simulink model "Quadcopter_Control_PID_Block_Updated"  (R2023a)
settings: Solver=VariableStepAuto  StartTime=0.0  StopTime=10.0  RelTol=1e-3
undefined symbols (not defined in the file or in its folder): sigbuilder_block
libraries: slpidlib x4
settings Model: Creator=Hameed  LastModifiedBy=Hameed
settings DebuggingCC: UnconnectedInputMsg=warning  UnconnectedOutputMsg=warning  UnconnectedLineMsg=warning
settings ModelReferenceCC: EnableRefExpFcnMdlSchedulingChecks=on
settings RTWCC: DLArmComputeVersion=19.05

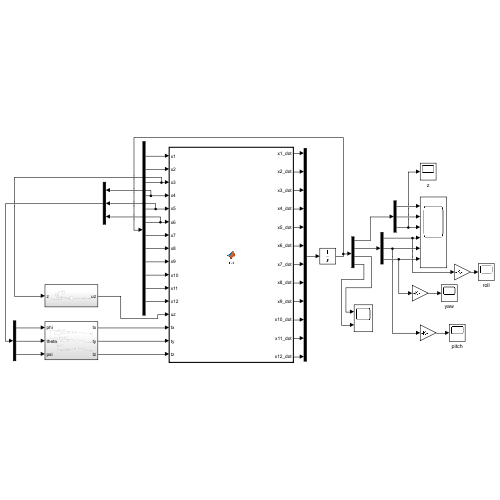
[thumbnail: Simulink's stored preview of the top-level diagram]
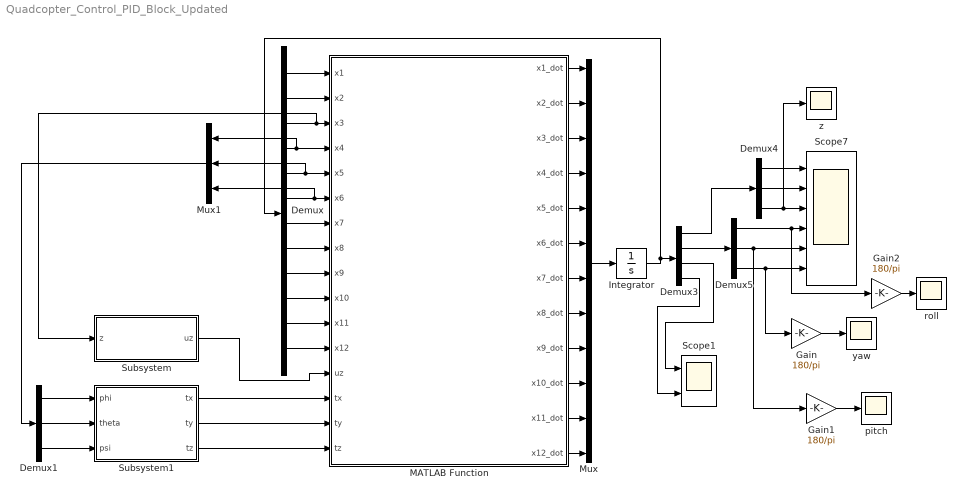
== system Quadcopter_Control_PID_Block_Updated ==
  Demux : Demux  Outputs=12
  Demux1 : Demux  Outputs=3
  Demux3 : Demux
  Demux4 : Demux  Outputs=3
  Demux5 : Demux  Outputs=3
  Gain : Gain  Gain=180/pi
  Gain1 : Gain  Gain=180/pi
  Gain2 : Gain  Gain=180/pi
  Integrator : Integrator  InitialCondition=[0;0;0;0;0;0;0;0;0;0;0;0]
  MATLAB Function : MATLAB Function  TreatAsAtomicUnit=on
  Mux : Mux  Inputs=12
  Mux1 : Mux  Inputs=3
  Scope1 : Scope  NumInputPorts=2
  Scope7 : Scope  NumInputPorts=6
  Subsystem : Subsystem
  Subsystem1 : Subsystem
  pitch : Scope
  roll : Scope
  yaw : Scope
  z : Scope
  wires:
  Demux3/1 -> Demux4/1
  Demux5/1 -> Gain2/1, Scope7/4
  MATLAB Function/9(x9_dot) -> Mux/9
  Demux/6 -> Mux1/3, MATLAB Function/6(x6)
  Demux/9 -> MATLAB Function/9(x9)
  Demux/10 -> MATLAB Function/10(x10)
  Demux1/3 -> Subsystem1/3(psi)
  Demux3/3 -> Scope1/1
  MATLAB Function/1(x1_dot) -> Mux/1
  Mux1/1 -> Demux1/1
  Integrator/1 -> Demux/1, Demux3/1
  Demux5/3 -> Gain/1, Scope7/6
  MATLAB Function/10(x10_dot) -> Mux/10
  Subsystem1/2(ty) -> MATLAB Function/15(ty)
  Demux/12 -> MATLAB Function/12(x12)
  Demux/11 -> MATLAB Function/11(x11)
  Demux/1 -> MATLAB Function/1(x1)
  Demux1/2 -> Subsystem1/2(theta)
  Demux/3 -> Subsystem/1(z), MATLAB Function/3(x3)
  MATLAB Function/3(x3_dot) -> Mux/3
  Mux/1 -> Integrator/1
  MATLAB Function/7(x7_dot) -> Mux/7
  Subsystem1/1(tx) -> MATLAB Function/14(tx)
  MATLAB Function/4(x4_dot) -> Mux/4
  Demux/4 -> MATLAB Function/4(x4), Mux1/1
  Subsystem/1(uz) -> MATLAB Function/13(uz)
  Demux3/2 -> Demux5/1
  MATLAB Function/2(x2_dot) -> Mux/2
  Demux/8 -> MATLAB Function/8(x8)
  Demux4/1 -> Scope7/1
  Subsystem1/3(tz) -> MATLAB Function/16(tz)
  Demux4/2 -> Scope7/2
  MATLAB Function/8(x8_dot) -> Mux/8
  Gain2/1 -> roll/1
  MATLAB Function/6(x6_dot) -> Mux/6
  Demux5/2 -> Gain1/1, Scope7/5
  Demux/7 -> MATLAB Function/7(x7)
  MATLAB Function/5(x5_dot) -> Mux/5
  Demux3/4 -> Scope1/2
  MATLAB Function/12(x12_dot) -> Mux/12
  Demux/5 -> Mux1/2, MATLAB Function/5(x5)
  MATLAB Function/11(x11_dot) -> Mux/11
  Demux1/1 -> Subsystem1/1(phi)
  Demux/2 -> MATLAB Function/2(x2)
  Gain/1 -> yaw/1
  Gain1/1 -> pitch/1
  Demux4/3 -> z/1, Scope7/3

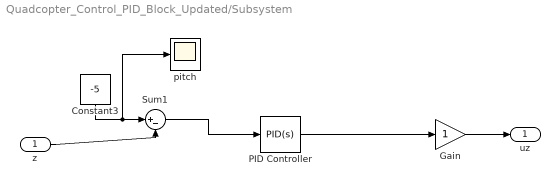
== system Quadcopter_Control_PID_Block_Updated/Subsystem ==
  z : Inport
  Constant3 : Constant  Value=-5
  Gain : Gain
  PID Controller : slpidlib/PID Controller  Controller=PID  Form=Parallel  TimeDomain=Continuous-time  UseExternalTs=off  SampleTime=-1  IntegratorMethod=Forward Euler  FilterMethod=Forward Euler  ControllerParametersSource=internal  P=-38.834932011976  I=-19.0341648234085  UseKiTs=off  D=-19.7761504332038  N=1142.8279760416  UseFilter=on  TunerSelectOption=Transfer Function Based (PID Tuner App)  InitialConditionSource=internal  InitialConditionForIntegrator=0  InitialConditionForFilter=0  DifferentiatorICPrevScaledInput=0  ExternalReset=none  TrackingMode=off  Kt=1  LimitOutput=off  SatLimitsSource=internal  UpperSaturationLimit=inf  LowerSaturationLimit=-inf  LinearizeAsGain=on  AntiWindupMode=none  Kb=1  LimitIntegrator=off  UpperIntegratorSaturationLimit=inf  LowerIntegratorSaturationLimit=-inf  POutMin=[]  POutMax=[]  IOutMin=[]  IOutMax=[]  DOutMin=[]  DOutMax=[]  NOutMin=[]  NOutMax=[]  SumOutMin=[]  SumOutMax=[]  SaturationOutMin=[]  SaturationOutMax=[]  PParamMin=[]  PParamMax=[]  IParamMin=[]  IParamMax=[]  DParamMin=[]  DParamMax=[]  NParamMin=[]  NParamMax=[]  KbParamMin=[]  KbParamMax=[]  KtParamMin=[]  KtParamMax=[]  KbOutMin=[]  KbOutMax=[]  KtOutMin=[]  KtOutMax=[]  IntegratorOutMin=[]  IntegratorOutMax=[]  FilterOutMin=[]  FilterOutMax=[]  SumI1OutMin=[]  SumI1OutMax=[]  SumI2OutMin=[]  SumI2OutMax=[]  SumI3OutMin=[]  SumI3OutMax=[]  SumI4OutMin=[]  SumI4OutMax=[]  SumDOutMin=[]  SumDOutMax=[]  DifferentiatorOutMin=[]  DifferentiatorOutMax=[]  FilterDiffOutCoefMin=[]  FilterDiffOutCoefMax=[]  ReciprocalOutMin=[]  ReciprocalOutMax=[]  SumDenOutMin=[]  SumDenOutMax=[]  SumNumOutMin=[]  SumNumOutMax=[]  DivideOutMin=[]  DivideOutMax=[]  UdiffTsProdOutMin=[]  UdiffTsProdOutMax=[]  NTsProdOutMin=[]  NTsProdOutMax=[]  UintegralTsProdOutMin=[]  UintegralTsProdOutMax=[]  UngainTsProdOutMin=[]  UngainTsProdOutMax=[]  ClampingZeroOutDataTypeStr=Inherit: Inherit via back propagation  ClampingZeroOutMin=[]  ClampingZeroOutMax=[]  FilterDenConstantOutDataTypeStr=Inherit: Inherit via back propagation  FilterDenConstantOutMin=[]  FilterDenConstantOutMax=[]  PCopyOutDataTypeStr=Inherit: Inherit via back propagation  PCopyOutMin=[]  PCopyOutMax=[]  NCopyOutDataTypeStr=Inherit: Inherit via back propagation  NCopyOutMin=[]  NCopyOutMax=[]  IntegratorContinuousStateAttributes=''  IntegratorStateMustResolveToSignalObject=off  IntegratorRTWStateStorageClass=Auto  FilterContinuousStateAttributes=''  FilterStateMustResolveToSignalObject=off  FilterRTWStateStorageClass=Auto  ParallelPVariant=InternalParameters  IdealPVariant=Disabled  IVariant=InternalParameters  DVariant=InternalParameters  IntegratorVariant=Continuous  SatVariant=Disabled  AWVariant=Passthrough  PCopyVariant=Disabled  TRVariant=Disabled  FdbkBlocksVariant=Forward  IdealPFdbkVariant=Disabled  SatFdbkVariant=Disabled  DerivativeFilterVariant=ContFilter  NVariant=InternalParameters  NCopyVariant=Disabled  FilterICVariant=InternalICsFilter  IntegratorICVariant=InternalICs  ExternalResetVariant=Disabled  TRSumVariant=Passthrough  SumFdbkVariant=Disabled  SumVariant=Sum_PID  TsampFilterVariant=InternalTs  TsampNgainVariant=Passthrough  TsampIntegralVariant=Disabled_SignalSpec  ExternalSaturationOutDataTypeStr=Inherit: Same as second input
  Sum1 : Sum  Inputs=|+-
  pitch : Scope
  uz : Outport
  wires:
  Gain/1 -> uz/1
  z/1 -> Sum1/2
  Constant3/1 -> pitch/1, Sum1/1
  PID Controller/1 -> Gain/1
  Sum1/1 -> PID Controller/1

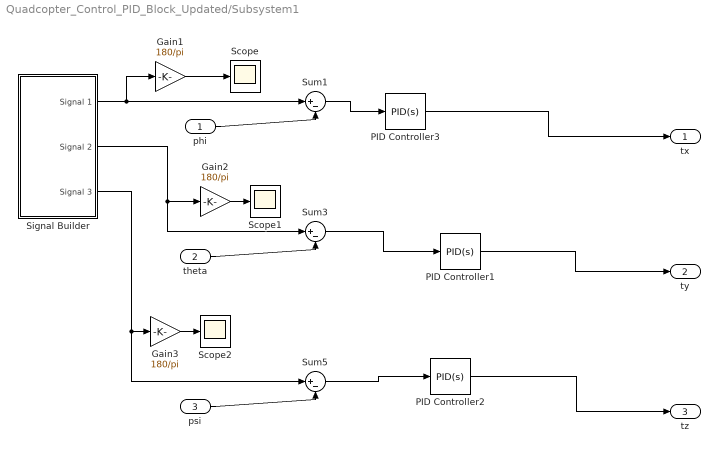
== system Quadcopter_Control_PID_Block_Updated/Subsystem1 ==
  phi : Inport
  theta : Inport  Port=2
  psi : Inport  Port=3
  Gain1 : Gain  Gain=180/pi
  Gain2 : Gain  Gain=180/pi
  Gain3 : Gain  Gain=180/pi
  PID Controller1 : slpidlib/PID Controller  Controller=PID  Form=Parallel  TimeDomain=Continuous-time  UseExternalTs=off  SampleTime=-1  IntegratorMethod=Forward Euler  FilterMethod=Forward Euler  ControllerParametersSource=internal  P=0.184522020618023  I=0.0815828774456371  UseKiTs=off  D=0.0909802954269596  N=76.1208933394499  UseFilter=on  TunerSelectOption=Transfer Function Based (PID Tuner App)  InitialConditionSource=internal  InitialConditionForIntegrator=0  InitialConditionForFilter=0  DifferentiatorICPrevScaledInput=0  ExternalReset=none  TrackingMode=off  Kt=1  LimitOutput=off  SatLimitsSource=internal  UpperSaturationLimit=inf  LowerSaturationLimit=-inf  LinearizeAsGain=on  AntiWindupMode=none  Kb=1  LimitIntegrator=off  UpperIntegratorSaturationLimit=inf  LowerIntegratorSaturationLimit=-inf  POutMin=[]  POutMax=[]  IOutMin=[]  IOutMax=[]  DOutMin=[]  DOutMax=[]  NOutMin=[]  NOutMax=[]  SumOutMin=[]  SumOutMax=[]  SaturationOutMin=[]  SaturationOutMax=[]  PParamMin=[]  PParamMax=[]  IParamMin=[]  IParamMax=[]  DParamMin=[]  DParamMax=[]  NParamMin=[]  NParamMax=[]  KbParamMin=[]  KbParamMax=[]  KtParamMin=[]  KtParamMax=[]  KbOutMin=[]  KbOutMax=[]  KtOutMin=[]  KtOutMax=[]  IntegratorOutMin=[]  IntegratorOutMax=[]  FilterOutMin=[]  FilterOutMax=[]  SumI1OutMin=[]  SumI1OutMax=[]  SumI2OutMin=[]  SumI2OutMax=[]  SumI3OutMin=[]  SumI3OutMax=[]  SumI4OutMin=[]  SumI4OutMax=[]  SumDOutMin=[]  SumDOutMax=[]  DifferentiatorOutMin=[]  DifferentiatorOutMax=[]  FilterDiffOutCoefMin=[]  FilterDiffOutCoefMax=[]  ReciprocalOutMin=[]  ReciprocalOutMax=[]  SumDenOutMin=[]  SumDenOutMax=[]  SumNumOutMin=[]  SumNumOutMax=[]  DivideOutMin=[]  DivideOutMax=[]  UdiffTsProdOutMin=[]  UdiffTsProdOutMax=[]  NTsProdOutMin=[]  NTsProdOutMax=[]  UintegralTsProdOutMin=[]  UintegralTsProdOutMax=[]  UngainTsProdOutMin=[]  UngainTsProdOutMax=[]  ClampingZeroOutDataTypeStr=Inherit: Inherit via back propagation  ClampingZeroOutMin=[]  ClampingZeroOutMax=[]  FilterDenConstantOutDataTypeStr=Inherit: Inherit via back propagation  FilterDenConstantOutMin=[]  FilterDenConstantOutMax=[]  PCopyOutDataTypeStr=Inherit: Inherit via back propagation  PCopyOutMin=[]  PCopyOutMax=[]  NCopyOutDataTypeStr=Inherit: Inherit via back propagation  NCopyOutMin=[]  NCopyOutMax=[]  IntegratorContinuousStateAttributes=''  IntegratorStateMustResolveToSignalObject=off  IntegratorRTWStateStorageClass=Auto  FilterContinuousStateAttributes=''  FilterStateMustResolveToSignalObject=off  FilterRTWStateStorageClass=Auto  ParallelPVariant=InternalParameters  IdealPVariant=Disabled  IVariant=InternalParameters  DVariant=InternalParameters  IntegratorVariant=Continuous  SatVariant=Disabled  AWVariant=Passthrough  PCopyVariant=Disabled  TRVariant=Disabled  FdbkBlocksVariant=Forward  IdealPFdbkVariant=Disabled  SatFdbkVariant=Disabled  DerivativeFilterVariant=ContFilter  NVariant=InternalParameters  NCopyVariant=Disabled  FilterICVariant=InternalICsFilter  IntegratorICVariant=InternalICs  ExternalResetVariant=Disabled  TRSumVariant=Passthrough  SumFdbkVariant=Disabled  SumVariant=Sum_PID  TsampFilterVariant=InternalTs  TsampNgainVariant=Passthrough  TsampIntegralVariant=Disabled_SignalSpec  ExternalSaturationOutDataTypeStr=Inherit: Same as second input
  PID Controller2 : slpidlib/PID Controller  Controller=PID  Form=Parallel  TimeDomain=Continuous-time  UseExternalTs=off  SampleTime=-1  IntegratorMethod=Forward Euler  FilterMethod=Forward Euler  ControllerParametersSource=internal  P=0.184522020618023  I=0.0815828774456371  UseKiTs=off  D=0.0909802954269596  N=76.1208933394499  UseFilter=on  TunerSelectOption=Transfer Function Based (PID Tuner App)  InitialConditionSource=internal  InitialConditionForIntegrator=0  InitialConditionForFilter=0  DifferentiatorICPrevScaledInput=0  ExternalReset=none  TrackingMode=off  Kt=1  LimitOutput=off  SatLimitsSource=internal  UpperSaturationLimit=inf  LowerSaturationLimit=-inf  LinearizeAsGain=on  AntiWindupMode=none  Kb=1  LimitIntegrator=off  UpperIntegratorSaturationLimit=inf  LowerIntegratorSaturationLimit=-inf  POutMin=[]  POutMax=[]  IOutMin=[]  IOutMax=[]  DOutMin=[]  DOutMax=[]  NOutMin=[]  NOutMax=[]  SumOutMin=[]  SumOutMax=[]  SaturationOutMin=[]  SaturationOutMax=[]  PParamMin=[]  PParamMax=[]  IParamMin=[]  IParamMax=[]  DParamMin=[]  DParamMax=[]  NParamMin=[]  NParamMax=[]  KbParamMin=[]  KbParamMax=[]  KtParamMin=[]  KtParamMax=[]  KbOutMin=[]  KbOutMax=[]  KtOutMin=[]  KtOutMax=[]  IntegratorOutMin=[]  IntegratorOutMax=[]  FilterOutMin=[]  FilterOutMax=[]  SumI1OutMin=[]  SumI1OutMax=[]  SumI2OutMin=[]  SumI2OutMax=[]  SumI3OutMin=[]  SumI3OutMax=[]  SumI4OutMin=[]  SumI4OutMax=[]  SumDOutMin=[]  SumDOutMax=[]  DifferentiatorOutMin=[]  DifferentiatorOutMax=[]  FilterDiffOutCoefMin=[]  FilterDiffOutCoefMax=[]  ReciprocalOutMin=[]  ReciprocalOutMax=[]  SumDenOutMin=[]  SumDenOutMax=[]  SumNumOutMin=[]  SumNumOutMax=[]  DivideOutMin=[]  DivideOutMax=[]  UdiffTsProdOutMin=[]  UdiffTsProdOutMax=[]  NTsProdOutMin=[]  NTsProdOutMax=[]  UintegralTsProdOutMin=[]  UintegralTsProdOutMax=[]  UngainTsProdOutMin=[]  UngainTsProdOutMax=[]  ClampingZeroOutDataTypeStr=Inherit: Inherit via back propagation  ClampingZeroOutMin=[]  ClampingZeroOutMax=[]  FilterDenConstantOutDataTypeStr=Inherit: Inherit via back propagation  FilterDenConstantOutMin=[]  FilterDenConstantOutMax=[]  PCopyOutDataTypeStr=Inherit: Inherit via back propagation  PCopyOutMin=[]  PCopyOutMax=[]  NCopyOutDataTypeStr=Inherit: Inherit via back propagation  NCopyOutMin=[]  NCopyOutMax=[]  IntegratorContinuousStateAttributes=''  IntegratorStateMustResolveToSignalObject=off  IntegratorRTWStateStorageClass=Auto  FilterContinuousStateAttributes=''  FilterStateMustResolveToSignalObject=off  FilterRTWStateStorageClass=Auto  ParallelPVariant=InternalParameters  IdealPVariant=Disabled  IVariant=InternalParameters  DVariant=InternalParameters  IntegratorVariant=Continuous  SatVariant=Disabled  AWVariant=Passthrough  PCopyVariant=Disabled  TRVariant=Disabled  FdbkBlocksVariant=Forward  IdealPFdbkVariant=Disabled  SatFdbkVariant=Disabled  DerivativeFilterVariant=ContFilter  NVariant=InternalParameters  NCopyVariant=Disabled  FilterICVariant=InternalICsFilter  IntegratorICVariant=InternalICs  ExternalResetVariant=Disabled  TRSumVariant=Passthrough  SumFdbkVariant=Disabled  SumVariant=Sum_PID  TsampFilterVariant=InternalTs  TsampNgainVariant=Passthrough  TsampIntegralVariant=Disabled_SignalSpec  ExternalSaturationOutDataTypeStr=Inherit: Same as second input
  PID Controller3 : slpidlib/PID Controller  Controller=PID  Form=Parallel  TimeDomain=Continuous-time  UseExternalTs=off  SampleTime=-1  IntegratorMethod=Forward Euler  FilterMethod=Forward Euler  ControllerParametersSource=internal  P=0.184522020618023  I=0.0815828774456371  UseKiTs=off  D=0.0909802954269596  N=76.1208933394499  UseFilter=on  TunerSelectOption=Transfer Function Based (PID Tuner App)  InitialConditionSource=internal  InitialConditionForIntegrator=0  InitialConditionForFilter=0  DifferentiatorICPrevScaledInput=0  ExternalReset=none  TrackingMode=off  Kt=1  LimitOutput=off  SatLimitsSource=internal  UpperSaturationLimit=inf  LowerSaturationLimit=-inf  LinearizeAsGain=on  AntiWindupMode=none  Kb=1  LimitIntegrator=off  UpperIntegratorSaturationLimit=inf  LowerIntegratorSaturationLimit=-inf  POutMin=[]  POutMax=[]  IOutMin=[]  IOutMax=[]  DOutMin=[]  DOutMax=[]  NOutMin=[]  NOutMax=[]  SumOutMin=[]  SumOutMax=[]  SaturationOutMin=[]  SaturationOutMax=[]  PParamMin=[]  PParamMax=[]  IParamMin=[]  IParamMax=[]  DParamMin=[]  DParamMax=[]  NParamMin=[]  NParamMax=[]  KbParamMin=[]  KbParamMax=[]  KtParamMin=[]  KtParamMax=[]  KbOutMin=[]  KbOutMax=[]  KtOutMin=[]  KtOutMax=[]  IntegratorOutMin=[]  IntegratorOutMax=[]  FilterOutMin=[]  FilterOutMax=[]  SumI1OutMin=[]  SumI1OutMax=[]  SumI2OutMin=[]  SumI2OutMax=[]  SumI3OutMin=[]  SumI3OutMax=[]  SumI4OutMin=[]  SumI4OutMax=[]  SumDOutMin=[]  SumDOutMax=[]  DifferentiatorOutMin=[]  DifferentiatorOutMax=[]  FilterDiffOutCoefMin=[]  FilterDiffOutCoefMax=[]  ReciprocalOutMin=[]  ReciprocalOutMax=[]  SumDenOutMin=[]  SumDenOutMax=[]  SumNumOutMin=[]  SumNumOutMax=[]  DivideOutMin=[]  DivideOutMax=[]  UdiffTsProdOutMin=[]  UdiffTsProdOutMax=[]  NTsProdOutMin=[]  NTsProdOutMax=[]  UintegralTsProdOutMin=[]  UintegralTsProdOutMax=[]  UngainTsProdOutMin=[]  UngainTsProdOutMax=[]  ClampingZeroOutDataTypeStr=Inherit: Inherit via back propagation  ClampingZeroOutMin=[]  ClampingZeroOutMax=[]  FilterDenConstantOutDataTypeStr=Inherit: Inherit via back propagation  FilterDenConstantOutMin=[]  FilterDenConstantOutMax=[]  PCopyOutDataTypeStr=Inherit: Inherit via back propagation  PCopyOutMin=[]  PCopyOutMax=[]  NCopyOutDataTypeStr=Inherit: Inherit via back propagation  NCopyOutMin=[]  NCopyOutMax=[]  IntegratorContinuousStateAttributes=''  IntegratorStateMustResolveToSignalObject=off  IntegratorRTWStateStorageClass=Auto  FilterContinuousStateAttributes=''  FilterStateMustResolveToSignalObject=off  FilterRTWStateStorageClass=Auto  ParallelPVariant=InternalParameters  IdealPVariant=Disabled  IVariant=InternalParameters  DVariant=InternalParameters  IntegratorVariant=Continuous  SatVariant=Disabled  AWVariant=Passthrough  PCopyVariant=Disabled  TRVariant=Disabled  FdbkBlocksVariant=Forward  IdealPFdbkVariant=Disabled  SatFdbkVariant=Disabled  DerivativeFilterVariant=ContFilter  NVariant=InternalParameters  NCopyVariant=Disabled  FilterICVariant=InternalICsFilter  IntegratorICVariant=InternalICs  ExternalResetVariant=Disabled  TRSumVariant=Passthrough  SumFdbkVariant=Disabled  SumVariant=Sum_PID  TsampFilterVariant=InternalTs  TsampNgainVariant=Passthrough  TsampIntegralVariant=Disabled_SignalSpec  ExternalSaturationOutDataTypeStr=Inherit: Same as second input
  Scope : Scope
  Scope1 : Scope
  Scope2 : Scope
  Signal Builder : Subsystem  Tag=STV Subsys  LoadFcn=sigbuilder_block('load');  StartFcn=sigbuilder_block('start');  StopFcn=sigbuilder_block('stop');  ClipboardFcn=sigbuilder_block('clipboard');  mask(Sigbuilder block){tuvar=[0:10]}
      mask help: Simulink:masks:SigbuilderBlock_MD
      mask init:
      | if ~strcmp(get_param(bdroot(gcbh),'SimulationStatus'),'stopped') tuvar = sigbuilder_block('maskInit'); end
      settings: CopyFcn=sigbuilder_block('copy');  DeleteFcn=sigbuilder_block('delete');  ModelCloseFcn=sigbuilder_block('modelClose');  PreSaveFcn=sigbuilder_block('preSave');  PauseFcn=sigbuilder_block('pause');  ContinueFcn=sigbuilder_block('continue');  NameChangeFcn=sigbuilder_block('namechange');  OpenFcn=sigbuilder_block('open',[437.6 153 550.4 359.25 ]);  CloseFcn=sigbuilder_block('close');
      mask Display: plot(0, 0, 100, 100,[2, 2, 32, 32, 2], [68, 8, 8, 68, 68],[32, 2], [38, 38], [32, 19, 2],[53, 60, 44], [32, 17, 17, 2],[16, 16, 31, 31]);txt = getActiveGroup(gcbh);text(2, 100, txt,'verticalAlignment', 'top');
  Sum1 : Sum  Inputs=|+-
  Sum3 : Sum  Inputs=|+-
  Sum5 : Sum  Inputs=|+-
  tx : Outport
  ty : Outport  Port=2
  tz : Outport  Port=3
  wires:
  Signal Builder/2(Signal 2) -> Sum3/1, Gain2/1
  phi/1 -> Sum1/2
  theta/1 -> Sum3/2
  psi/1 -> Sum5/2
  Sum1/1 -> PID Controller3/1
  PID Controller3/1 -> tx/1
  Sum3/1 -> PID Controller1/1
  PID Controller1/1 -> ty/1
  Sum5/1 -> PID Controller2/1
  PID Controller2/1 -> tz/1
  Signal Builder/1(Signal 1) -> Sum1/1, Gain1/1
  Signal Builder/3(Signal 3) -> Gain3/1, Sum5/1
  Gain1/1 -> Scope/1
  Gain2/1 -> Scope1/1
  Gain3/1 -> Scope2/1

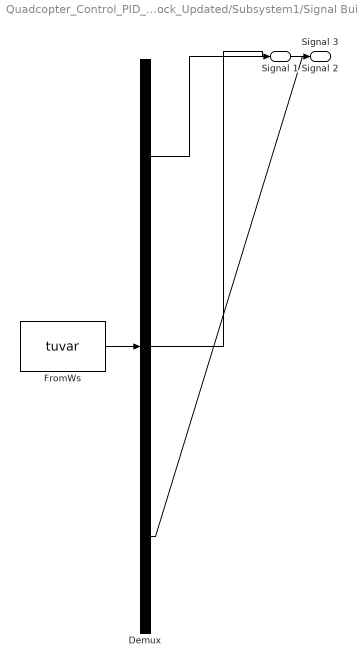
== system Quadcopter_Control_PID_Block_Updated/Subsystem1/Signal Builder ==
  Demux : Demux  Tag=STV Demux  Outputs=3
      settings: DisplayOption=none
  FromWs : FromWorkspace  Tag=STV FromWs  VariableName=tuvar
      SigBuilderData=|
      | common.afterFinalStr = 'Extrapolate'
      | common.sampleTime = 0
      | dataSet.timeRange = [0 30]
      | dataSet.name = 'Group 1'
      | sbobj.Groups.Name = 'Group 1'
      | sbobj.Groups.Signals(1).Name = 'Signal 1'
      | sbobj.Groups.Signals(1).XData = [0 6 6 10 10 30]
      | sbobj.Groups.Signals(1).YData = [0 0 0.349065850399 0.349065850399 0 0]
      | sbobj.Groups.Signals(2).Name = 'Signal 2'
      | sbobj.Groups.Signals(2).XData = [0 14 14 18 18 30]
      | sbobj.Groups.Signals(2).YData = [0 0 0.261799387799 0.261799387799 0 0]
      | sbobj.Groups.Signals(3).Name = 'Signal 3'
      | sbobj.Groups.Signals(3).XData = [0 22 22 26 26 30]
      | sbobj.Groups.Signals(3).YData = [0 0 0.785398163397 0.785398163397 0 0]
      | sbobj.Groups.TimeRange = [0 30]
  Signal 1 : Outport  Tag=STV Outport
  Signal 2 : Outport  Tag=STV Outport  Port=2
  Signal 3 : Outport  Tag=STV Outport  Port=3
  wires:
  Demux/1 -> Signal 1/1
  FromWs/1 -> Demux/1
  Demux/2 -> Signal 2/1
  Demux/3 -> Signal 3/1

== matlab function Quadcopter_Control_PID_Block_Updated/MATLAB Function ==
  data: x1 input; x1_dot output; x2 input; x3 input; x4 input; x5 input; x6 input; x7 input; x8 input; x9 input; x10 input; x11 input; x12 input; x2_dot output; x3_dot output; x4_dot output; x5_dot output; x6_dot output; x7_dot output; x8_dot output; x9_dot output; x10_dot output; x11_dot output; x12_dot output; uz input; tx input; ty input; tz input
function [x1_dot,x2_dot,x3_dot,x4_dot,x5_dot,x6_dot,x7_dot,x8_dot,x9_dot,x10_dot,x11_dot,x12_dot]= fcn(x1,x2,x3,x4,x5,x6,x7,x8,x9,x10,x11,x12,uz,tx,ty,tz)

% Ixx= 1.2; 
% Iyy= 1.2;
% Izz= 0.3;
%Izz= 2.3;
%k=1;
k = 1e-3;
L= 0.25;
m= 2;
%km= 0.2;
%km = 0.5e-4;
g= 9.81;
%gamma = km/k; 

Ixx = (1/12)*m*(0.2^2+0.2^2);
Iyy= (1/12)*m*(0.2^2+0.2^2);
Izz= (1/12)*m*(0.2^2+0.2^2);
I= [Ixx 0 0;0 Iyy 0;0 0 Izz];


%R-ZYX Euler
R = [cos(x5)*cos(x6), sin(x4)*sin(x5)*cos(x6)-cos(x4)*sin(x6), cos(x4)*sin(x5)*cos(x6)+sin(x4)*sin(x6);
     cos(x5)*sin(x6), sin(x4)*sin(x5)*sin(x6)+cos(x4)*cos(x6), cos(x4)*sin(x5)*sin(x6)-sin(x4)*cos(x6);
     -sin(x5), sin(x4)*cos(x5), cos(x4)*cos(x5)];


Q = [1 0 -sin(x5);
     0 cos(x4) cos(x5)*sin(x4);
     0 -sin(x4) cos(x5)*cos(x4)];

dQ = [0 0 -cos(x5);
      0 -sin(x4) -sin(x5)*sin(x4)+cos(x5)*cos(x4);
      0 -cos(x4) -sin(x5)*cos(x4)-cos(x5)*sin(x4)];

%P=Q';
%  P=[1 0 0; 
%     0 cos(x4) -sin(x4); 
%     -sin(x5) cos(x5)*sin(x4) cos(x5)*cos(x4)];
%  
 
 
 
M = Q'.*I*Q;

ndot=[x10;x11;x12];

s = Q*ndot;
S = [0 -s(3) s(2);s(3) 0 -s(1);-s(2) s(1) 0];
C = Q'.*S*I*Q + Q'.*I*dQ;

%%-------------------------------------------------------------------

%%---------------------------------------------------

% A = [ 1 1 1 1;
%       0  L 0 -L;
%      -L 0  L  0;
%      gamma -gamma gamma -gamma];
 
%  A = [ 0 0 0 0;
%       0 0 0 0;
%       1 1 1 1;
%       0  L 0 -L;
%      -L 0  L  0;
%      gamma -gamma gamma -gamma];

% 
% %references
% xd = 0; yd = 0; zd = -2;
% phid = pi/4.; thetad = pi/4.; psid = pi/4.;
% 
% %error signals
% ez = zd-x3;
% ephi = phid-x4;
% etheta = thetad-x5;
% epsi = psid-x6;
% 
% %controller
% 
% uz = -(50*ez-60*x9);
% tx = (1*ephi-2*x10);
% ty = (1*etheta-2*x11);
% tz = (1*epsi-2*x12);


%  u = [uz;tx;ty;tz];
%  %u = [0;0;uz;tx;ty;tz];
%  th = pinv(A)*u;
%  w = (th/k);         % actually it's omeega square
% %w= sqrt(th/k);
% % %u=k*A*ws;


 T = uz;
 tB = [tx;ty;tz];

%T = k*(w(1)+w(2)+w(3)+w(4));
%T = k*(w(1)^2+w(2)^2+w(3)^2+w(4)^2);

%tB= [L*k*(w(2)-w(4));L*k*(-w(1)+w(3));km*(w(1)-w(2)+w(3)-w(4))];
%tB= [L*k*(w(2)^2-w(4)^2);L*k*(-w(1)^2+w(3)^2);km*(w(1)^2-w(2)^2+w(3)^2-w(4)^2)];


%Jinv=inv(J)
%x789= g*[0;0;1]-R*[0;0;T]/m;


x789 = (1/m)*(-R*[0;0;T]+ m*g*[0;0;1]);
%x789 = (1/m)*(-k*R*A(1:3,:)*w+ m*g*[0;0;1] );


%x101112 = pinv(M)*(tB-C*ndot);
x101112 = pinv(M)*(Q'*tB-C*ndot);


x1_dot=x7;
x2_dot=x8;
x3_dot=x9;

x4_dot=x10;
x5_dot=x11;
x6_dot=x12;

x7_dot=x789(1);
x8_dot=x789(2);
x9_dot=x789(3);

x10_dot=x101112(1);
x11_dot=x101112(2);
x12_dot=x101112(3);


%%-----------------------------------------------------------------------------













%%-------------------------------------------------------------------------------


% C11=0;
% C12=(Iyy-Izz)*(x11*cos(x4)*sin(x4)+x12*sin(x4)^2*cos(x5))+(Izz-Iyy)*x12*cos(x4)^2*cos(x5)-Ixx*x12*cos(x5);
% C13=(Izz-Iyy)*(x12*cos(x4)*sin(x4)*cos(x5)^2);
% C21=(Izz-Iyy)*(x11*cos(x4)*sin(x4)+x12*sin(x4)*cos(x5))+(Iyy-Izz)*x12*cos(x4)^2*cos(x5)+Ixx*x12*cos(x5);
% C22=(Izz-Iyy)*x10*cos(x4)*sin(x4);
% C23= -Ixx*x12*sin(x5)*cos(x5)+Iyy*x12*sin(x4)^2*sin(x5)*cos(x5)+ Izz*x12*cos(x4)^2*sin(x5)*cos(x5);
% C31=(Iyy-Izz)*(x12*cos(x5)^2*sin(x4)*cos(x4))-Ixx*x11*cos(x5);
% C32= (Izz-Iyy)*(x11*cos(x4)*sin(x4)*sin(x5)+x10*sin(x4)^2*cos(x5))+(Iyy-Izz)*x10*cos(x4)^2*cos(x5)+Ixx*x12*sin(x5)*cos(x5)-Iyy*x12*sin(x10)^2*sin(x5)*cos(x5)-Izz*x12*cos(x10)^2*sin(x5)*cos(x5);
% C33=(Iyy-Izz)*x10*cos(x4)*sin(x4)*cos(x5)^2-Iyy*x11*sin(x4)^2*cos(x5)*sin(x5)-Izz*x11*cos(x4)^2*cos(x5)*sin(x5)+Ixx*x11*cos(x5)*sin(x5);
% C=[C11 C12 C13;C21 C22 C23;C31 C32 C33];
